simulink model "Lab_3"  (Simulink 9.2)
settings: Solver=VariableStepAuto  StartTime=0.0  StopTime=simulation_time  RelTol=10e-13  AbsTol=10e-14
values from neighbouring files (symbols this model uses):
  a = (r_a + r_p)/2    (= 7178)    [main.m]
  A_BN_0 = eye(3)    [main.m]
  i = 0    [main.m]
  I = [I_1,   0,  0 ... (first row only)    [main.m]
  I_inv = inv(I)    [main.m]
  mu = 398600    [main.m]
  OMG = 0    [main.m]
  omg = 0    [main.m]
  phi_0 = 0    [main.m]
  psi_0 = 0    [main.m]
  theta = 0    [main.m]
  theta_0 = 0    [main.m]
  w_0 = [w1_0,w2_0,w3_0]    [main.m]
undefined symbols (not defined in the file or in its folder): k1, k2
libraries: sharedutil x1
settings Model: Creator=fcuzzocrea  LastModifiedBy=fcuzzocrea
settings SolverCC: AutoScaleAbsTol=off
settings DataIOCC: LimitDataPoints=off  SaveFormat=Dataset  SignalLoggingSaveFormat=Dataset
settings OptimizationCC: LifeSpan=auto
settings DebuggingCC: UnderspecifiedInitializationDetection=Simplified  MergeDetectMultiDrivingBlocksExec=error  FcnCallInpInsideContextMsg=error  StateNameClashWarn=none  LibraryContextMissingDiagnostic=none  SFUnexpectedBacktrackingDiag=error  SFNoUnconditionalDefaultTransitionDiag=error  SFExecutionAtInitializationDiag=warning
settings HardwareCC: ProdBitPerPointer=64  ProdBitPerSizeT=64  ProdBitPerPtrDiffT=64  ProdLargestAtomicFloat=Float  ProdIntDivRoundTo=Zero  ProdEndianess=LittleEndian  ProdWordSize=64  ProdHWDeviceType=Intel->x86-64 (Windows64)
settings ModelReferenceCC: PropagateSignalLabelsOutOfModel=on
settings CodeAppCC: StateflowObjectComments=off
settings GRTTargetCC: TargetLangStandard=C99 (ISO)  GeneratePreprocessorConditionals=Use local settings  CombineOutputUpdateFcns=on  GRTInterface=off
settings ConfigComp: CovMetricSettings=dwe  CovHtmlReporting=off  CovSaveCumulativeToWorkspaceVar=off  CovSaveSingleToWorkspaceVar=off  CovExternalEMLEnable=on

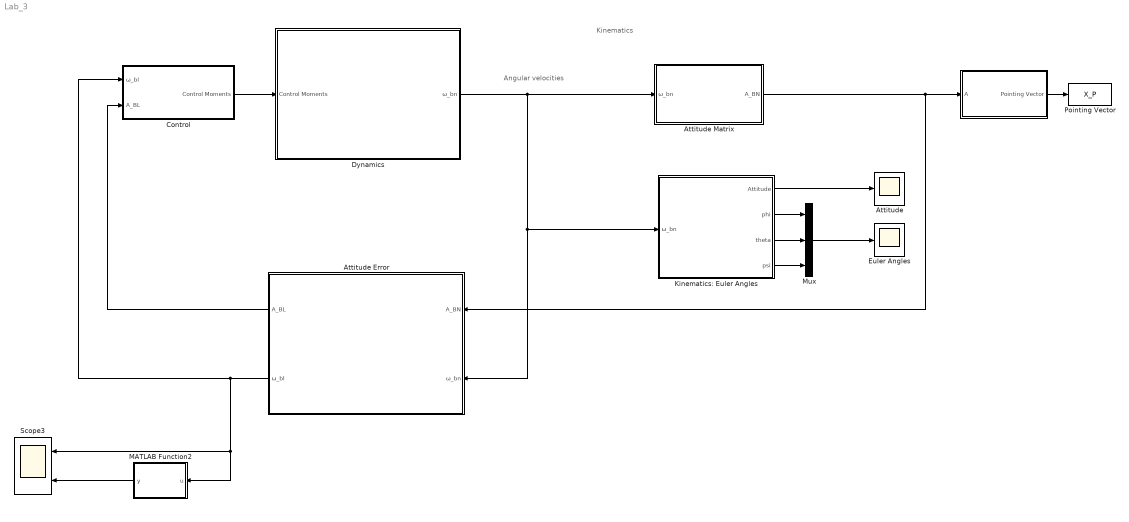
== system Lab_3 ==
  note: Kinematics
  note: Angular velocities
  " " : Subsystem
  Attitude : Scope
  Attitude Error : Subsystem
  Attitude Matrix : Subsystem
  Control : Subsystem
  "Dynamics  " : Subsystem
  Euler Angles : Scope
  Kinematics: Euler Angles : Subsystem
  MATLAB Function2 : MATLAB Function  TreatAsAtomicUnit=on
  Mux : Mux  Inputs=3
  "Pointing Vector " : ToWorkspace  VariableName=X_P  SampleTime=-1
  Scope3 : Scope  NumInputPorts=2
  wires:
  Attitude Matrix/1(A_BN) -> Attitude Error/1(A_BN), " "/1(A)
  " "/1("Pointing Vector ") -> "Pointing Vector "/1
  Kinematics: Euler Angles/1(Attitude) -> Attitude/1
  "Dynamics  "/1(ω_bn) -> Attitude Error/2(ω_bn), Kinematics: Euler Angles/1(ω_bn), Attitude Matrix/1(ω_bn)
  Attitude Error/1(A_BL) -> Control/2(A_BL)
  Kinematics: Euler Angles/3(theta) -> Mux/2
  Kinematics: Euler Angles/4(psi) -> Mux/3
  Kinematics: Euler Angles/2(phi) -> Mux/1
  Mux/1 -> Euler Angles/1
  Attitude Error/2(ω_bl) -> MATLAB Function2/1(u), Scope3/1, Control/1(ω_bl)
  MATLAB Function2/1(y) -> Scope3/2
  Control/1(Control Moments) -> "Dynamics  "/1(Control Moments)

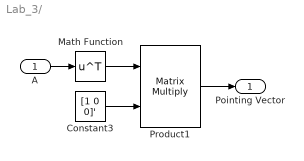
== system Lab_3/  ==
  A : Inport
  Constant3 : Constant  Value=[1 0 0]'  VectorParams1D=off
  Math Function : Math  Operator=transpose  SaturateOnIntegerOverflow=on
  Product1 : Product  Multiplication=Matrix(*)
  "Pointing Vector " : Outport
  wires:
  Constant3/1 -> Product1/2
  Math Function/1 -> Product1/1
  A/1 -> Math Function/1
  Product1/1 -> "Pointing Vector "/1

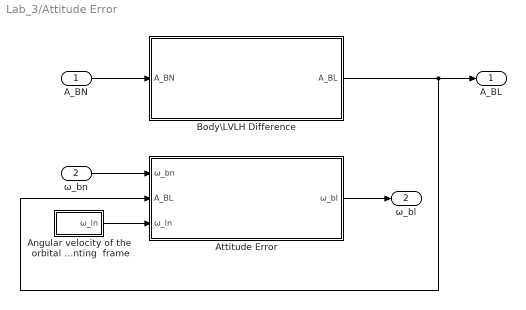
== system Lab_3/Attitude Error ==
  A_BN : Inport
  ω_bn : Inport  Port=2
  Angular velocity of the  orbital pointing  frame : Subsystem
  Attitude Error : Subsystem
  Body\LVLH Difference : Subsystem
  A_BL : Outport
  ω_bl : Outport  Port=2
  wires:
  A_BN/1 -> Body\LVLH Difference/1("A_BN ")
  ω_bn/1 -> Attitude Error/1(ω_bn)
  Body\LVLH Difference/1("A_BL   ") -> A_BL/1, Attitude Error/2("A_BL ")
  Angular velocity of the  orbital pointing  frame/1(ω_ln) -> Attitude Error/3("ω_ln ")
  Attitude Error/1(ω_bl) -> ω_bl/1

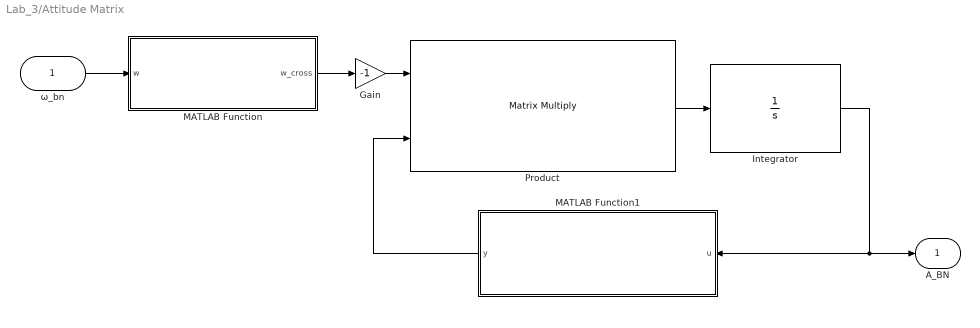
== system Lab_3/Attitude Matrix ==
  ω_bn : Inport  Unit=rad/s  PortDimensions=3
  Gain : Gain  Gain=-1
  Integrator : Integrator  InitialCondition=A_BN_0
  MATLAB Function : MATLAB Function  TreatAsAtomicUnit=on
  MATLAB Function1 : MATLAB Function  TreatAsAtomicUnit=on
  Product : Product  Multiplication=Matrix(*)
  A_BN : Outport
  wires:
  Product/1 -> Integrator/1
  MATLAB Function/1(w_cross) -> Gain/1
  Integrator/1 -> A_BN/1, MATLAB Function1/1(u)
  ω_bn/1 -> MATLAB Function/1(w)
  Gain/1 -> Product/1
  MATLAB Function1/1(y) -> Product/2

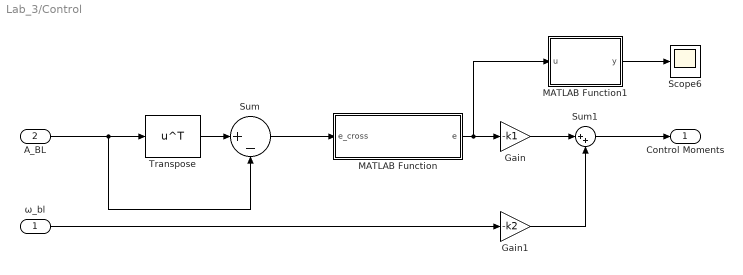
== system Lab_3/Control ==
  ω_bl : Inport
  A_BL : Inport  Port=2
  Gain : Gain  Gain=-k1
  Gain1 : Gain  Gain=-k2
  MATLAB Function : MATLAB Function  TreatAsAtomicUnit=on
  MATLAB Function1 : MATLAB Function  TreatAsAtomicUnit=on
  Scope6 : Scope
  Sum : Sum  Inputs=|+-
  Sum1 : Sum  Inputs=|++
  Transpose : Math  Operator=transpose  SaturateOnIntegerOverflow=on
  Control Moments : Outport
  wires:
  Gain/1 -> Sum1/1
  Gain1/1 -> Sum1/2
  A_BL/1 -> Sum/2, Transpose/1
  ω_bl/1 -> Gain1/1
  Sum1/1 -> Control Moments/1
  MATLAB Function1/1(y) -> Scope6/1
  Transpose/1 -> Sum/1
  MATLAB Function/1(e) -> Gain/1, MATLAB Function1/1(u)
  Sum/1 -> MATLAB Function/1(e_cross)

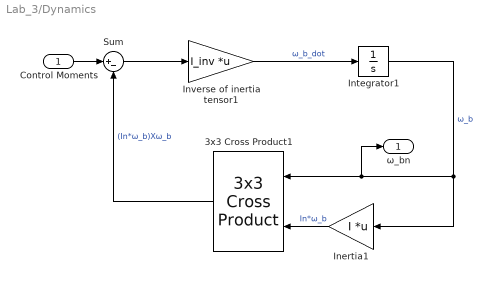
== system Lab_3/Dynamics   ==
  Control Moments : Inport
  3x3 Cross Product1 : sharedutil/3x3 Cross Product  aMode=aMode
      settings: SourceProductBaseCode=AE
  Inertia1 : Gain  Gain=I  Multiplication=Matrix(K*u)
  Integrator1 : Integrator  InitialCondition=w_0
  Inverse of inertia tensor1 : Gain  Gain=I_inv  Multiplication=Matrix(K*u)
  Sum : Sum  Inputs=|+-
  ω_bn : Outport
  wires:
  Inertia1/1 -> 3x3 Cross Product1/2  "In*ω_b"
  Inverse of inertia tensor1/1 -> Integrator1/1  "ω_b_dot"
  3x3 Cross Product1/1 -> Sum/2  "(In*ω_b)Xω_b"
  Integrator1/1 -> Inertia1/1, 3x3 Cross Product1/1, ω_bn/1  "ω_b"
  Sum/1 -> Inverse of inertia tensor1/1
  Control Moments/1 -> Sum/1

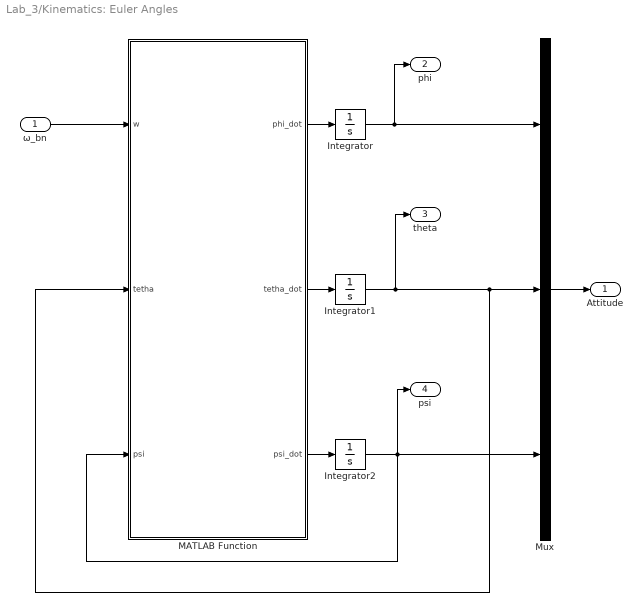
== system Lab_3/Kinematics: Euler Angles ==
  ω_bn : Inport
  Integrator : Integrator  InitialCondition=phi_0
  Integrator1 : Integrator  InitialCondition=theta_0
  Integrator2 : Integrator  InitialCondition=psi_0
  MATLAB Function : MATLAB Function  TreatAsAtomicUnit=on
  Mux : Mux  Inputs=3
  Attitude : Outport
  phi : Outport  Port=2
  theta : Outport  Port=3
  psi : Outport  Port=4
  wires:
  Integrator2/1 -> MATLAB Function/3(psi), Mux/3, psi/1
  Mux/1 -> Attitude/1
  Integrator1/1 -> MATLAB Function/2(tetha), Mux/2, theta/1
  Integrator/1 -> Mux/1, phi/1
  MATLAB Function/3(psi_dot) -> Integrator2/1
  MATLAB Function/2(tetha_dot) -> Integrator1/1
  MATLAB Function/1(phi_dot) -> Integrator/1
  ω_bn/1 -> MATLAB Function/1(w)

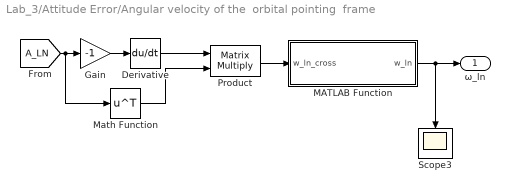
== system Lab_3/Attitude Error/Angular velocity of the  orbital pointing  frame ==
  Derivative : Derivative
  Gain : Gain  Gain=-1
  MATLAB Function : MATLAB Function  TreatAsAtomicUnit=on
  Math Function : Math  Operator=transpose  SaturateOnIntegerOverflow=on
  Product : Product  Multiplication=Matrix(*)
  Scope3 : Scope
  ω_ln : Outport
  wires:
  Math Function/1 -> Product/2
  Derivative/1 -> Product/1
  Product/1 -> MATLAB Function/1(w_ln_cross)
  MATLAB Function/1(w_ln) -> ω_ln/1, Scope3/1
  [A_LN] -> Gain/1, Math Function/1
  Gain/1 -> Derivative/1

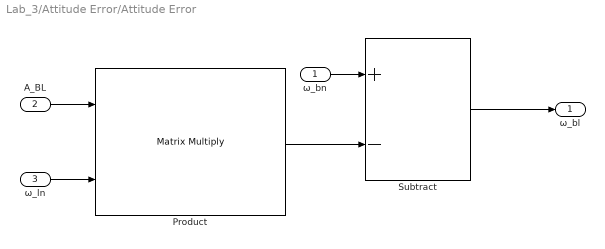
== system Lab_3/Attitude Error/Attitude Error ==
  ω_bn : Inport
  "A_BL " : Inport  Port=2
  "ω_ln " : Inport  Port=3
  Product : Product  Multiplication=Matrix(*)
  Subtract : Sum  Inputs=+-
  ω_bl : Outport
  wires:
  Product/1 -> Subtract/2
  Subtract/1 -> ω_bl/1
  ω_bn/1 -> Subtract/1
  "A_BL "/1 -> Product/1
  "ω_ln "/1 -> Product/2

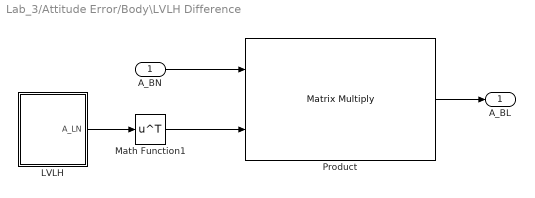
== system Lab_3/Attitude Error/Body\LVLH Difference ==
  "A_BN " : Inport
  LVLH : Subsystem
  Math Function1 : Math  Operator=transpose  SaturateOnIntegerOverflow=on
  Product : Product  Multiplication=Matrix(*)
  "A_BL   " : Outport
  wires:
  "A_BN "/1 -> Product/1
  Product/1 -> "A_BL   "/1
  Math Function1/1 -> Product/2
  LVLH/1("A_LN ") -> Math Function1/1

== system Lab_3/Attitude Error/Body\LVLH Difference/LVLH ==
  Full Orbital Dynamics : Subsystem
  Initial Conditions (KEP) : Constant  Value=[a, e, i, OMG, omg, theta]
  Planetary Constant : Constant  Value=mu
  "A_LN " : Outport
  tag scope: A_LN=global
  wires:
  Planetary Constant/1 -> Full Orbital Dynamics/1(mu)
  Initial Conditions (KEP)/1 -> Full Orbital Dynamics/2(Initial Condition (kep))
  Full Orbital Dynamics/1(A_LN) -> [A_LN], "A_LN "/1

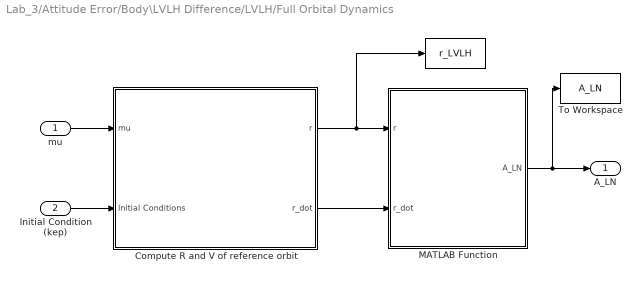
== system Lab_3/Attitude Error/Body\LVLH Difference/LVLH/Full Orbital Dynamics ==
  mu : Inport
  Initial Condition (kep) : Inport  Port=2
  "  " : ToWorkspace  VariableName=r_LVLH  SampleTime=-1
  Compute R and V of reference orbit : Subsystem
  MATLAB Function : MATLAB Function  TreatAsAtomicUnit=on
  To Workspace : ToWorkspace  VariableName=A_LN  SampleTime=-1
  A_LN : Outport
  wires:
  mu/1 -> Compute R and V of reference orbit/1(mu)
  Initial Condition (kep)/1 -> Compute R and V of reference orbit/2(Initial Conditions)
  Compute R and V of reference orbit/1(r) -> "  "/1, MATLAB Function/1(r)
  MATLAB Function/1(A_LN) -> To Workspace/1, A_LN/1
  Compute R and V of reference orbit/2(r_dot) -> MATLAB Function/2(r_dot)

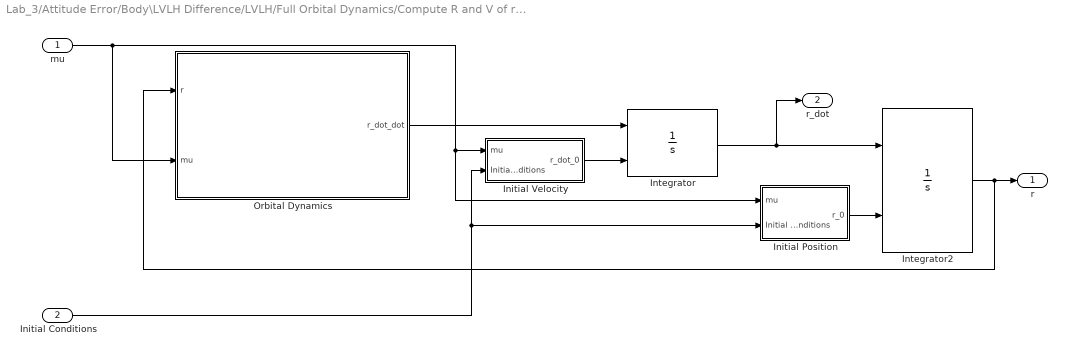
== system Lab_3/Attitude Error/Body\LVLH Difference/LVLH/Full Orbital Dynamics/Compute R and V of reference orbit ==
  mu : Inport
  Initial Conditions : Inport  Port=2
  Initial Position : Subsystem
  Initial Velocity : Subsystem
  Integrator : Integrator  InitialConditionSource=external  InitialCondition=[r,v]=kep2car(kep,mu);  ContinuousStateAttributes='velocity'
  Integrator2 : Integrator  InitialConditionSource=external  InitialCondition=[r,v]=kep2car(kep,mu);  ContinuousStateAttributes='position'
  Orbital Dynamics : MATLAB Function  TreatAsAtomicUnit=on
  r : Outport
  r_dot : Outport  Port=2
  wires:
  Initial Conditions/1 -> Initial Position/2(Initial Conditions), Initial Velocity/2(Initial Conditions)
  Initial Position/1(r_0) -> Integrator2/2
  Initial Velocity/1(r_dot_0) -> Integrator/2
  Orbital Dynamics/1(r_dot_dot) -> Integrator/1
  Integrator/1 -> r_dot/1, Integrator2/1
  mu/1 -> Initial Position/1(mu), Initial Velocity/1(mu), Orbital Dynamics/2(mu)
  Integrator2/1 -> Orbital Dynamics/1(r), r/1

== system Lab_3/Attitude Error/Body\LVLH Difference/LVLH/Full Orbital Dynamics/Compute R and V of reference orbit/Initial Position ==
  mu : Inport
  Initial Conditions : Inport  Port=2
  MATLAB Function2 : MATLAB Function  TreatAsAtomicUnit=on
  r_0 : Outport
  wires:
  MATLAB Function2/1(r_0) -> r_0/1
  mu/1 -> MATLAB Function2/2(mu)
  Initial Conditions/1 -> MATLAB Function2/1(kep)

== system Lab_3/Attitude Error/Body\LVLH Difference/LVLH/Full Orbital Dynamics/Compute R and V of reference orbit/Initial Velocity ==
  mu : Inport
  Initial Conditions : Inport  Port=2
  MATLAB Function1 : MATLAB Function  TreatAsAtomicUnit=on
  r_dot_0 : Outport
  wires:
  MATLAB Function1/1(r_dot_0) -> r_dot_0/1
  mu/1 -> MATLAB Function1/2(mu)
  Initial Conditions/1 -> MATLAB Function1/1(kep)

== matlab function Attitude Matrix/MATLAB Function ==
  data: w input double; w_cross output double
function w_cross  = assembly_w_cross(w)

w_cross = [0, -w(3), w(2);
           w(3), 0, -w(1);
          -w(2), w(1), 0];

== matlab function Attitude Matrix/MATLAB Function1 ==
  data: u input double; y output double
function y = ortonormalize(u)
%#codegen
% Ortonormalize a matrix.
% Reference : Lecture 7, Slide 5 SADC Polimi

y = u.*3/2 - u*u'*(u./2);

y = u;

end

== matlab function Control/MATLAB Function ==
  data: e_cross input double; e output double
function e = e_extractor(e_cross)

e_1 = e_cross(3,2);
e_2 = e_cross(1,3);
e_3 = e_cross(2,1);

e = [e_1, e_2, e_3]';
end

== matlab function Control/MATLAB Function1 ==
  data: u input double; y output double
function y = fcn(u)

y = norm(u);

== matlab function MATLAB Function2 ==
  data: u input double; y output double
function y = fcn(u)

y = norm(u);

== matlab function Kinematics: Euler Angles/MATLAB Function ==
  data: phi_dot output double; tetha_dot output double; psi_dot output double; w input double; tetha input double; psi input double
function [phi_dot,tetha_dot, psi_dot] = euler_eqtns(w, tetha, psi)

% Euler rotations (sequence 123)
%phi_dot = 1/cos(tetha)*((w(1)*cos(psi)-w(2)*sin(psi)));
%tetha_dot = (w(2)*cos(psi))+(w(1)*sin(psi));
%psi_dot = w(3) - ((w(1)*cos(psi) - w(2)*sin(psi))*(sin(tetha)/cos(tetha)));

% Euler rotations (sequence 321)
phi_dot = 1/cos(tetha)*(w(2)*sin(psi) + w(3)*cos(psi));

tetha_dot = (w(2)*cos(psi)-w(3)*sin(psi));

psi_dot = w(1) + 1/cos(tetha)*(w(2)*sin(tetha)*sin(psi) + w(3)*sin(tetha)*cos(psi)); 

end

== matlab function Attitude Error/Angular velocity of the orbital pointing frame/MATLAB Function ==
  data: w_ln_cross input double; w_ln output double
function w_ln = w_component_extractor(w_ln_cross)

w_1 = w_ln_cross(3,2);
w_2 = w_ln_cross(1,3);
w_3 = w_ln_cross(2,1);

w_ln = [w_1, w_2, w_3]';
end

== matlab function Attitude Error/Body\LVLH Difference/LVLH/Full Orbital Dynamics/Compute R and V of reference orbit/Initial Position/MATLAB Function2 ==
  data: r_0 output double; kep input double; mu input double
function r_0  = kep2car(kep,mu)

% Using kep2car function to find position and velocity at initial condition
[r_0,~]=kep2car(kep,mu);

end

== matlab function Attitude Error/Body\LVLH Difference/LVLH/Full Orbital Dynamics/Compute R and V of reference orbit/Initial Velocity/MATLAB Function1 ==
  data: r_dot_0 output double; kep input double; mu input double
function r_dot_0  = kep2car(kep,mu)

% Using kep2car function to find velocity at initial condition
[~,r_dot_0]=kep2car(kep,mu);

end

== matlab function Attitude Error/Body\LVLH Difference/LVLH/Full Orbital Dynamics/Compute R and V of reference orbit/Orbital Dynamics ==
  data: r input double; r_dot_dot output double; mu input double
function r_dot_dot  = orbit_equation(r,mu)

r_dot_dot = -(mu/norm(r)^3)*r;

end

== matlab function Attitude Error/Body\LVLH Difference/LVLH/Full Orbital Dynamics/MATLAB Function ==
  data: r input double; A_LN output double; r_dot input double
function A_LN = assembly_A_LN(r,r_dot)
% This M-Function builds an LVLH frame from a position vector and a 
% velocity vector

r = r';
r_dot = r_dot';

o_1 = -r/norm(r);                                       % Points toward the Earth, aligned with S/C - Earth direction (x)
o_3 = -(cross(r,r_dot))/(norm(cross(r,r_dot)));         % Points in the direction of angular momentum vector (z)
o_2 = cross(o_3,o_1);                                   % Points into the direction of the motion (y)
     
A_LN = [o_1; o_2; o_3];

end
